simulink model "drone_test"  (R2022a)
settings: Solver=VariableStepAuto  StartTime=0.0  StopTime=600  RelTol=1e-3
values from neighbouring files (symbols this model uses):
  D = [Env.UnrealRiverPts(Env.RiverRegions(i,4),1) Env.UnrealRiverPts(Env.RiverRegions(i,4),2)]    [DefineUAVPath.m]    (also in DistributeIceXML.m; DistributeIceXML1.m; DroneSurveyRegions.m; EstimateIceNumerals.m)
libraries: sim3dlib x4, uavsim3dlib x2, sim3dcameralib x1, sim3dphyssensorlib x1, visionsinks x1
settings Model: Creator=zckog  LastModifiedBy=lab
settings DebuggingCC: UnconnectedInputMsg=warning  UnconnectedOutputMsg=warning  UnconnectedLineMsg=warning
settings RTWCC: DLArmComputeVersion=19.05

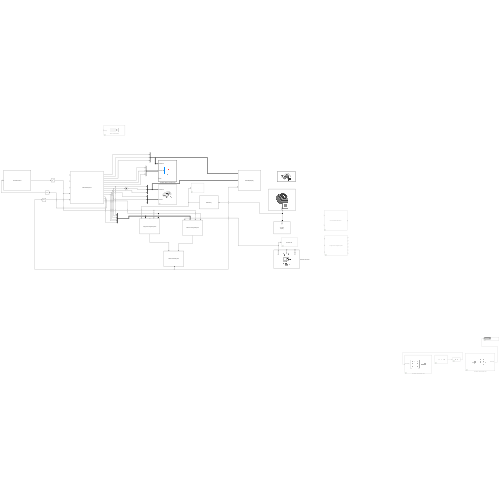
[thumbnail: Simulink's stored preview of the top-level diagram]
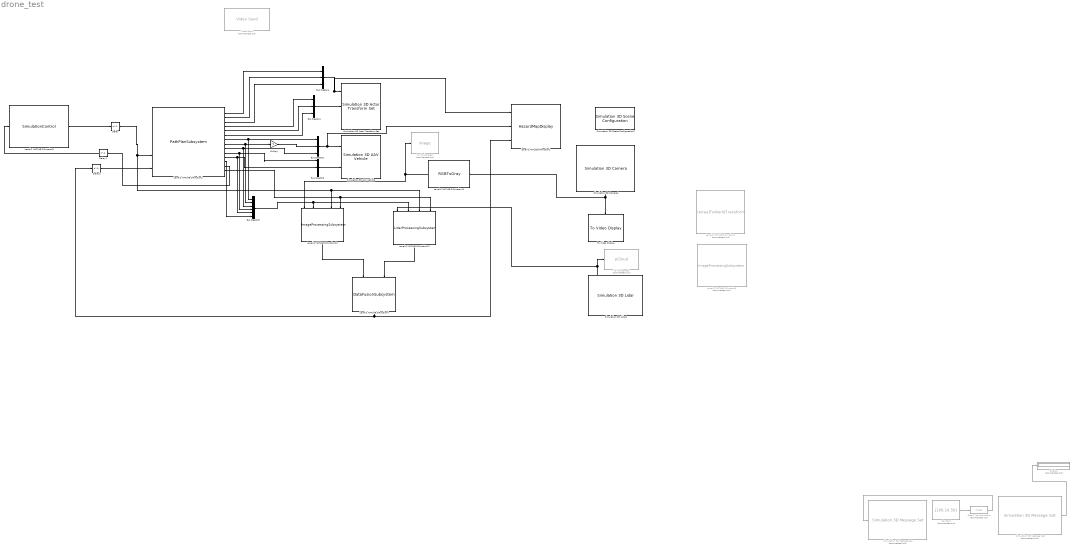
== system drone_test ==
  Bus Creator{1..4} (4 alike) : BusCreator  Inputs=3
  Bus Creator5 : BusCreator  Inputs=6
  Constant : Constant  Commented=on  Value=[100,10,50]  VectorParams1D=off  OutDataTypeStr=single
  Data Type Conversion : DataTypeConversion  Commented=on  OutDataTypeStr=single  SaturateOnIntegerOverflow=off  RndMeth=Floor
  Delay : Delay  DelayLength=1  InitialCondition=0
  Delay1 : Delay  DelayLength=1  InitialCondition=0
  Delay2 : Delay  DelayLength=1  InitialCondition=0
  Display : Display  Commented=on
  Level-2 MATLAB S-Function1 : M-S-Function  Priority=1  FunctionName=HazardMapDisplay
  Level-2 MATLAB S-Function10 : M-S-Function  Priority=1  FunctionName=ImageProcessingSubsystem
  Level-2 MATLAB S-Function11 : M-S-Function  Priority=1  FunctionName=RGBToGray
  Level-2 MATLAB S-Function12 : M-S-Function  Priority=1  FunctionName=LidarProcessingSubsystem
  Level-2 MATLAB S-Function2 : M-S-Function  Priority=1  FunctionName=PathPlanSubsystem
  Level-2 MATLAB S-Function3 : M-S-Function  Priority=1  Commented=on  FunctionName=UnrealToWorldTransform
  Level-2 MATLAB S-Function4 : M-S-Function  Priority=1  FunctionName=DataFusionSubsystem
  Level-2 MATLAB S-Function8 : M-S-Function  Priority=1  FunctionName=SimulationControl
  Level-2 MATLAB S-Function9 : M-S-Function  Priority=1  Commented=on  FunctionName=ImageProcessingSubsystem
  Multiply : Gain  Gain=-1
  Simulation 3D Actor Transform Set : sim3dlib/Simulation 3D Actor Transform Set  Priority=2  ActorTag=SimulinkActor1  NumberOfParts=1  CustNumOfParts=3  Translation=[0 0 0]  Rotation=[0 0 0]  Scale=[1 1 1]  Ts=-1  aMode=0
      settings: SourceProductBaseCode=VE,AE,DR,UV,VE
  Simulation 3D Camera1 : sim3dcameralib/Simulation 3D Camera  Priority=1  sensorTag=Sim3dSensor1  sensorId=1  sensorName=Sim3dSensor1  vehTagList={'Drone1';'Scene Origin'}  vehTag=Drone1  mountLoc=Origin  offsetFlag=on  tmountOffset=[0, 0, 0]  extTmount=off  rmountOffset=[0, 90, 90]  extRmount=off  FocalLength=[1109, 1109]  OpticalCenter=[640, 360]  ImageSize=[720, 1280]  RadialDistortion=[0, 0]  TangentialDistortion=[0, 0]  SensorSkew=0  DepthOutportEnabled=off  SemanticOutportEnabled=off  TransformOutportEnabled=off  SampleTime=-1  mountPoint=[0 0 0]  mountOrientation=[0 -90 -90]  aMode=3  ID=1
      settings: SourceProductBaseCode=VE,AE,DR,UV,VE
  Simulation 3D Lidar1 : sim3dphyssensorlib/Simulation 3D Lidar  Priority=1  sensorTag=Sim3dSensor3  sensorId=3  sensorName=Sim3dSensor3  vehTagList={'Drone1';'Scene Origin'}  vehTag=Drone1  mountLoc=Origin  offsetFlag=on  tmountOffset=[0, 0, 0]  rmountOffset=[0, 90,90]  DetectionRange=120  RangeResolution=0.002  VerticalFOV=33.75  VerticalResolution=1.6875  HorizontalFOV=60  HorizontalResolution=3  DistanceOutportEnabled=off  ReflectivityOutportEnabled=off  TransformOutportEnabled=on  SampleTime=-1  mountPoint=[0 0 0]  mountOrientation=[0 -90 -90]  aMode=4  ID=3
      settings: SourceProductBaseCode=VE,AE,DR,UV,VE
  Simulation 3D Message Get : sim3dlib/Simulation 3D Message Get  Priority=1  Commented=on  SigName=ConeLocGet  DataType=single  MsgSize=[1 3]  Ts=-1  aMode=0
      settings: SourceProductBaseCode=VE,AE,DR,UV,VE
  Simulation 3D Message Set : sim3dlib/Simulation 3D Message Set  Priority=-1  Commented=on  SigName=ConeLocSet  Ts=-1  aMode=0
      settings: SourceProductBaseCode=VE,AE,DR,UV,VE
  Simulation 3D Scene Configuration2 : sim3dlib/Simulation 3D Scene Configuration  Priority=1  ProjectFormat=Unreal Editor  SceneDesc=Straight road  ProjectName=D:\Matlab2021\toolbox\shared\sim3d_projects\automotive_project\UE4\WindowsNoEditor\VehicleSimulation.exe  ScenePath=/Game/Maps/HwStrght  UEProjPath=D:\OneDrive - York University\MASS\UNREALxMATLAB\UNREALxMATLAB\DroneExp1\DroneExp1\DroneExp1.uproject  vehTagList={'Drone1';'Scene Origin'}  vehTag=Scene Origin  OpVisEn=off  Ts=1/30  EnableWindow=on  EnableRemoteAccess=off  EnableWeather=off  SunAltitude=40.0  SunAzimuth=90  clouds=10  wind=1  fog=0  rain=0  sensorTag=MainCamera3  sensorId=3  sensorName=MainCamera3  mountLoc=Origin  offsetFlag=off  tmountOffset=[0, 0, 0]  rmountOffset=[0, 0, 0]  HorizontalResolution=1280  VerticalResolution=720  HorizontalFOV=60  mountPoint=[0 0 0]  mountOrientation=[0 0 0]  aMode=3  ID=3
      settings: SourceProductBaseCode=VE,AE,DR,UV,VE
  Simulation 3D UAV Vehicle : uavsim3dlib/Simulation 3D UAV Vehicle  Priority=2  Mesh=Quadrotor  MeshPath=/MathWorksUAVContent/UAVs/HexaRotorUAV/HexaRotor.HexaRotor  Color=Black  ActorName=Drone1  InitialTranslation=[0 0 0]  InitialRotation=[0 0 0]  SampleTime=-1  ActorType=SimulinkVehicle  ID=C  aMode=4  ActorTag=Drone1
      settings: SourceProductBaseCode=UV
  To Video Display : visionsinks/To Video Display  windowSizeMode=Normal  openAtMdlStart=on  fullScreen=off  videoWindowX=1  videoWindowY=31  saveWindowSize=off  videoWindowWidth=958  videoWindowHeight=1008  inputColorFormat=RGB  inputType=Obsolete  imagePorts=One multidimensional signal  OutputDevice=On-screen video monitor  dataOrg=Column-major  isWindowOpen=off
  To Workspace1 : ToWorkspace  Commented=on  VariableName=pCloud  SaveFormat=Timeseries  SampleTime=-1
  To Workspace8 : ToWorkspace  Commented=on  VariableName=image  SaveFormat=Timeseries  SampleTime=-1
  Video Send : uavsim3dlib/Video Send  Commented=on  ImageFormat=RGB  ImageSignal=One multidimensional signal  Compression=JPEG  JPEGQuality=85  VPXFrameDeadline=30  RemoteAddress=10.0.0.136  RemotePort=5004
      settings: SourceProductBaseCode=UV
  wires:
  Constant/1 -> Data Type Conversion/1
  Data Type Conversion/1 -> Simulation 3D Message Set/1
  Simulation 3D Message Get/1 -> Display/1
  Simulation 3D Camera1/1 -> To Video Display/1, Level-2 MATLAB S-Function11/1
  Level-2 MATLAB S-Function11/1 -> Level-2 MATLAB S-Function10/1, To Workspace8/1
  Level-2 MATLAB S-Function8/1 -> Delay/1
  Delay/1 -> Level-2 MATLAB S-Function2/4, Level-2 MATLAB S-Function10/4, Level-2 MATLAB S-Function12/3
  Level-2 MATLAB S-Function2/13 -> Delay1/1
  Delay1/1 -> Level-2 MATLAB S-Function8/1
  Level-2 MATLAB S-Function2/10 -> Bus Creator5/4, Bus Creator3/1
  Level-2 MATLAB S-Function2/11 -> Bus Creator5/5, Bus Creator3/2
  Level-2 MATLAB S-Function2/9 -> Bus Creator5/3, Bus Creator2/3
  Level-2 MATLAB S-Function2/8 -> Bus Creator5/2, Multiply/1
  Bus Creator2/1 -> Level-2 MATLAB S-Function1/2, Simulation 3D UAV Vehicle/1
  Multiply/1 -> Bus Creator2/2
  Bus Creator3/1 -> Simulation 3D UAV Vehicle/2
  Level-2 MATLAB S-Function2/14 -> Level-2 MATLAB S-Function10/5, Level-2 MATLAB S-Function12/4
  Bus Creator1/1 -> Level-2 MATLAB S-Function1/1, Simulation 3D Actor Transform Set/1
  Level-2 MATLAB S-Function2/1 -> Bus Creator1/1
  Level-2 MATLAB S-Function2/2 -> Bus Creator1/2
  Level-2 MATLAB S-Function2/3 -> Bus Creator1/3
  Level-2 MATLAB S-Function2/6 -> Bus Creator4/3
  Level-2 MATLAB S-Function2/4 -> Bus Creator4/1
  Level-2 MATLAB S-Function2/5 -> Bus Creator4/2
  Bus Creator4/1 -> Simulation 3D Actor Transform Set/2
  Simulation 3D Lidar1/1 -> Level-2 MATLAB S-Function12/1, To Workspace1/1
  Level-2 MATLAB S-Function2/7 -> Bus Creator2/1, Bus Creator5/1
  Level-2 MATLAB S-Function2/12 -> Bus Creator5/6
  Bus Creator5/1 -> Level-2 MATLAB S-Function12/2, Level-2 MATLAB S-Function10/2
  Delay2/1 -> Level-2 MATLAB S-Function2/5
  Level-2 MATLAB S-Function10/1 -> Level-2 MATLAB S-Function4/1
  Level-2 MATLAB S-Function12/1 -> Level-2 MATLAB S-Function4/2
  Level-2 MATLAB S-Function4/1 -> Level-2 MATLAB S-Function1/3, Delay2/1
